simulink model "test_KP"  (R2023b)
settings: Solver=VariableStepAuto  StartTime=0.0  StopTime=0.1  RelTol=1e-3
undefined symbols (not defined in the file or in its folder): testCase
libraries: nav_lib x2
settings Model: Creator=brent  LastModifiedBy=brent

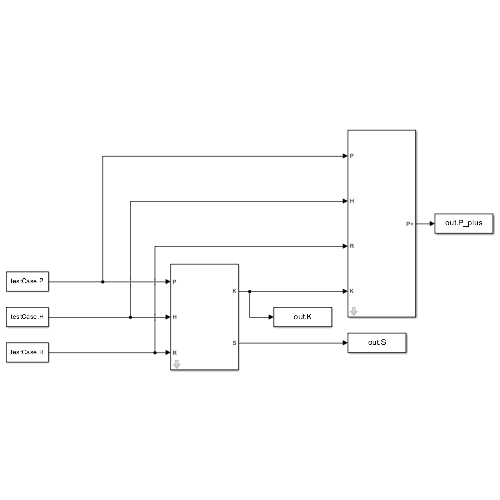
[thumbnail: Simulink's stored preview of the top-level diagram]
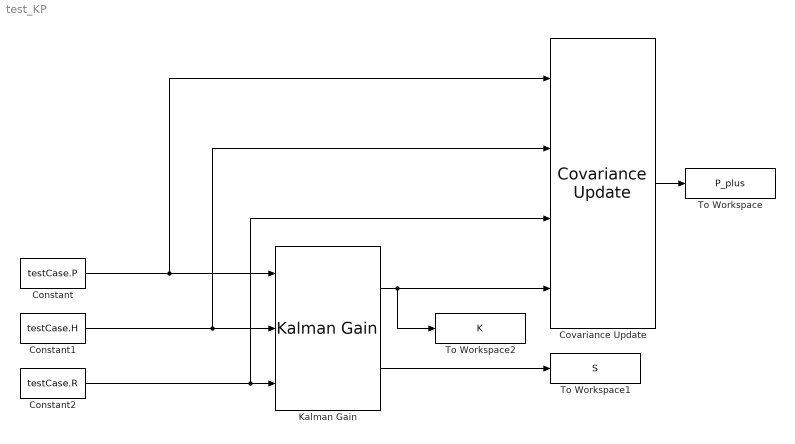
== system test_KP ==
  Constant : Constant  Value=testCase.P
  Constant1 : Constant  Value=testCase.H  VectorParams1D=off
  Constant2 : Constant  Value=testCase.R
  Covariance Update : nav_lib/Covariance Update
      settings: SourceProductName=Navigation library
  Kalman Gain : nav_lib/Kalman Gain
      settings: SourceProductName=Navigation library
  To Workspace : ToWorkspace  VariableName=P_plus  SampleTime=-1
  To Workspace1 : ToWorkspace  VariableName=S  SampleTime=-1
  To Workspace2 : ToWorkspace  VariableName=K  SampleTime=-1
  wires:
  Kalman Gain/1 -> To Workspace2/1, Covariance Update/4
  Constant1/1 -> Covariance Update/2, Kalman Gain/2
  Constant2/1 -> Covariance Update/3, Kalman Gain/3
  Constant/1 -> Covariance Update/1, Kalman Gain/1
  Covariance Update/1 -> To Workspace/1
  Kalman Gain/2 -> To Workspace1/1
